simulink model "uz_3ph_ParameterID"  (R2022b)
settings: Solver=FixedStepDiscrete  StartTime=0.0  StopTime=160  FixedStep=0.000005  RelTol=1e-3  EnableMultiTasking=on
model workspace (MATLAB code in the model file):
  | cmdLim = Simulink.Parameter;
  | cmdLim.Value = 15;
  | cmdLim.Description = 'Limit for controlling the maximum surface command angle.';
  | cmdLim.Min = 0;
  | cmdLim.Max = 90;
  | cmdLim.DocUnits = 'deg';
  | 
  | dispGain = Simulink.Parameter;
  | dispGain.Value = 0.75;
  | dispGain.Description = 'Gain applied to the displacement error.';
  | dispGain.Min = 0;
  | dispGain.Max = [];
  | dispGain.DocUnits = 'deg/sec/deg';
  | 
  | dispLim = Simulink.Parameter;
  | dispLim.Value = 30;
  | dispLim.Description = 'Limit for controlling the maximum commanded angle.';
  | dispLim.Min = 0;
  | dispLim.Max = 180;
  | dispLim.DocUnits = 'deg';
  | 
  | intGain = Simulink.Parameter;
  | intGain.Value = 0.5;
  | intGain.Description = 'Gain applied to the integral error.';
  | intGain.Min = 0;
  | intGain.Max = [];
  | intGain.DocUnits = 'deg/sec/deg/sec';
  | 
  | intLim = Simulink.Parameter;
  | intLim.Value = 5;
  | intLim.Description = 'Limit for controlling the maximum commanded angle.';
  | intLim.Min = 0;
  | intLim.Max = 90;
  | intLim.DocUnits = 'deg';
  | 
  | rateGain = Simulink.Parameter;
  | rateGain.Value = 2;
  | rateGain.Description = 'Gain applied to the rate error.';
  | rateGain.Min = 0;
  | rateGain.Max = [];
  | rateGain.DocUnits = 'deg/deg/sec';
  | 
  | rateLim = Simulink.Parameter;
  | rateLim.Value = 6;
  | rateLim.Description = 'Limit for controlling the maximum commanded angle.';
  | rateLim.Min = 0;
  | rateLim.Max = 180;
  | rateLim.DocUnits = 'deg/sec';
  | 
  | hdgGain = Simulink.Parameter;
  | hdgGain.Value = 0.015;
values from neighbouring files (symbols this model uses):
  d_d_TMS = 0.005    [Parameter_Init_Buehler_201.m]
  d_f_hardware = 200000    [Parameter_Init_Buehler_201.m]
  d_f_states = 20000    [Parameter_Init_Buehler_201.m]
  d_i_max = 15    [Parameter_Init_Buehler_201.m]
  d_i_min = -d_i_max    (= -15)    [Parameter_Init_Buehler_201.m]
  d_I_n = 8    [Parameter_Init_Buehler_201.m]
  d_J_Coupling_M_E = 2e-6    (= 2e-06)    [Parameter_Init_Buehler_201.m]
  d_J_Coupling_M_Ms = 2e-20    [Parameter_Init_Buehler_201.m]
  d_J_Ms_L = d_J_Ms_M    (= 1.26363648e-05)    [Parameter_Init_Buehler_201.m]
  d_J_Ms_M = 0.5*0.5*((0.5*d_d_Ms)^4)*3.14*d_l_Ms*d_rho_Ms    (= 1.26363648e-05)    [Parameter_Init_Buehler_201.m]
  d_L_d = 0.00031    [Parameter_Init_Buehler_201.m]
  d_L_q = 0.00033    [Parameter_Init_Buehler_201.m]
  d_p = 4    [Parameter_Init_Buehler_201.m]
  d_psi_pm = 0.0075    [Parameter_Init_Buehler_201.m]
  d_R_ph = d_R_ph_ph/2    (= 0.089)    [Parameter_Init_Buehler_201.m]
  d_y_max = 10    [Parameter_Init_Buehler_201.m]
  d_y_min = -d_y_max    (= -10)    [Parameter_Init_Buehler_201.m]
undefined symbols (not defined in the file or in its folder): i_dq, i_dq_ref, n_ref, V_abc, v_dq
libraries: fl_lib x47, nesl_utility x30, ee_lib x18, simulink x8, spsabctodq0Lib x2, spsdq0toabcLib x1, spsTriangleGeneratorLib x1
(part 2 of 4)

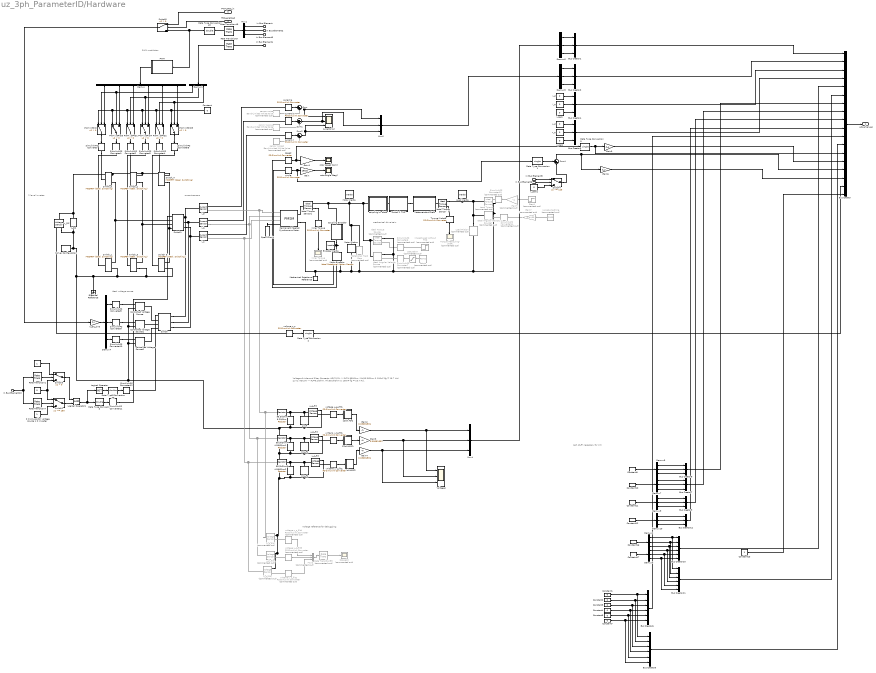
== system uz_3ph_ParameterID/Hardware ==
  note: 6ph stuff, necessary for init
  note: PWM modulator
  note: 2 level inverter
  note: current sensors
  note: ideal voltage source
  note: Voltage divider and filter:
      | Concerto: ADC 3,3V -> RL=4,99kOhm. Mit 95,3kOhm & 100nF (fg = 16,7 Hz).
      | Zynq: ADC 5V -> RL=8,2kOhm. Mit 95,3kOhm & 100nF (fg = 16,7 Hz).
  note: Voltage reference
      | for debugging:
  note: mechanical drive train
  In Bus Element : Inport  PortName=ElectricalID_output  Element=PWM_Switch_0
  In Bus Element2 : Inport  PortName=ElectricalID_output  Element=PWM_Switch_2
  In Bus Element3 : Inport  PortName=ElectricalID_output  Element=PWM_Switch_4
  In Bus Element4 : Inport  PortName=ElectricalID_output  Element=enable_TriState
  In Bus Element5 : Inport  PortName=ElectricalID_output  Element=thetaOffset
  In Bus Element10 : Inport  Port=2  PortName=ElectricalID_FOC_output  Element=activeState
  In Bus Element6 : Inport  Port=2  PortName=ElectricalID_FOC_output  Element=activeState
  PWM_FOC_in : Inport  Port=3
  FOC_enabled : Inport  Port=4
  " " : Constant  Value=0
  "   " : Constant
  "0 = sinusoidal voltage source 1 = inverter    " : Constant
  0.1µF1 : ee_lib/Passive/Capacitor  cap_option=0  c=47 nF  Cvec=[ 1e-5 1e-6 ] F  Vvec=[ 0 10 ] V  CV_table_symmetry=1  f_vec=[1, 10] kHz  DFext_vec=[.8, 1.2]  enable_C_tol=0  C_tol=0.1  tol_distribution=1  nSigma=4  r=1e-18 Ohm  g=0 1/Ohm  averaging_period=0 s  enable_operating_limits=0  operating_limit_action=2  max_working_voltage_range=[ -25 25 ] V  power_rating=1 W  enable_faults=0  fault_action=1  Cscale_faulted=100  R_faulted=0.001 Ohm  G_faulted=0 1/Ohm  tau_fault=0.001 s  enable_temporal_fault=0  t_fault=1 s  enable_behavioral_fault=0  max_permissible_voltage_range=[ -100 100 ] V  t_fail_on_voltage=1 s  i_specify=off  i_priority=None  i=0 A  i_nominal_specify=off  i_nominal_unit=A  i_nominal_value=1  v_specify=off  v_priority=None  v=0 V  v_nominal_specify=off  v_nominal_unit=V  v_nominal_value=1  vc_specify=on  vc_priority=High  vc=0 V  vc_nominal_specify=off  vc_nominal_unit=V  vc_nominal_value=1
  0.1µF2 : ee_lib/Passive/Capacitor  cap_option=0  c=47 nF  Cvec=[ 1e-5 1e-6 ] F  Vvec=[ 0 10 ] V  CV_table_symmetry=1  f_vec=[1, 10] kHz  DFext_vec=[.8, 1.2]  enable_C_tol=0  C_tol=0.1  tol_distribution=1  nSigma=4  r=1e-18 Ohm  g=0 1/Ohm  averaging_period=0 s  enable_operating_limits=0  operating_limit_action=2  max_working_voltage_range=[ -25 25 ] V  power_rating=1 W  enable_faults=0  fault_action=1  Cscale_faulted=100  R_faulted=0.001 Ohm  G_faulted=0 1/Ohm  tau_fault=0.001 s  enable_temporal_fault=0  t_fault=1 s  enable_behavioral_fault=0  max_permissible_voltage_range=[ -100 100 ] V  t_fail_on_voltage=1 s  i_specify=off  i_priority=None  i=0 A  i_nominal_specify=off  i_nominal_unit=A  i_nominal_value=1  v_specify=off  v_priority=None  v=0 V  v_nominal_specify=off  v_nominal_unit=V  v_nominal_value=1  vc_specify=on  vc_priority=High  vc=0 V  vc_nominal_specify=off  vc_nominal_unit=V  vc_nominal_value=1
  12bit ADC : MATLAB Function  TreatAsAtomicUnit=on
  12bit ADC1 : MATLAB Function  TreatAsAtomicUnit=on
  12bit ADC2 : MATLAB Function  TreatAsAtomicUnit=on
  4,99kOhm1 : ee_lib/Passive/Resistor  R=8200 Ohm  enable_R_tol=0  R_tol=0.1  tol_distribution=1  nSigma=4  enable_operating_limits=0  operating_limit_action=2  max_working_voltage=100 V  power_rating=1 W  enable_faults=0  fault_action=1  R_faulted=Inf Ohm  enable_temporal_fault=0  t_fault=1 s  enable_behavioral_fault=0  max_permissible_current=1 A  t_fail_on_current=1 s  noise_mode=0  sample_time=0.001 s  repeatability=1  auto_seed=3499211588  user_seed=0  Tdevice=25 degC  power_derating_T1=70 degC  power_derating_T2=155 degC  operating_temperature_range_vec=[-50, 150] degC  alpha=3.93e-3 1/K  Tmeas=25 degC  thermal_mass=100 J/K  temperature_specify=off  temperature_priority=High  temperature=298.15 K  temperature_nominal_specify=off  temperature_nominal_unit=K  temperature_nominal_value=1
  4,99kOhm2 : ee_lib/Passive/Resistor  R=8200 Ohm  enable_R_tol=0  R_tol=0.1  tol_distribution=1  nSigma=4  enable_operating_limits=0  operating_limit_action=2  max_working_voltage=100 V  power_rating=1 W  enable_faults=0  fault_action=1  R_faulted=Inf Ohm  enable_temporal_fault=0  t_fault=1 s  enable_behavioral_fault=0  max_permissible_current=1 A  t_fail_on_current=1 s  noise_mode=0  sample_time=0.001 s  repeatability=1  auto_seed=3890346746  user_seed=0  Tdevice=25 degC  power_derating_T1=70 degC  power_derating_T2=155 degC  operating_temperature_range_vec=[-50, 150] degC  alpha=3.93e-3 1/K  Tmeas=25 degC  thermal_mass=100 J/K  temperature_specify=off  temperature_priority=High  temperature=298.15 K  temperature_nominal_specify=off  temperature_nominal_unit=K  temperature_nominal_value=1
  47nF : ee_lib/Passive/Capacitor  cap_option=0  c=47 nF  Cvec=[ 1e-5 1e-6 ] F  Vvec=[ 0 10 ] V  CV_table_symmetry=1  f_vec=[1, 10] kHz  DFext_vec=[.8, 1.2]  enable_C_tol=0  C_tol=0.1  tol_distribution=1  nSigma=4  r=1e-20 Ohm  g=0 1/Ohm  averaging_period=0 s  enable_operating_limits=0  operating_limit_action=2  max_working_voltage_range=[ -25 25 ] V  power_rating=1 W  enable_faults=0  fault_action=1  Cscale_faulted=100  R_faulted=0.001 Ohm  G_faulted=0 1/Ohm  tau_fault=0.001 s  enable_temporal_fault=0  t_fault=1 s  enable_behavioral_fault=0  max_permissible_voltage_range=[ -100 100 ] V  t_fail_on_voltage=1 s  i_specify=off  i_priority=None  i=0 A  i_nominal_specify=off  i_nominal_unit=A  i_nominal_value=1  v_specify=off  v_priority=None  v=0 V  v_nominal_specify=off  v_nominal_unit=V  v_nominal_value=1  vc_specify=on  vc_priority=High  vc=0 V  vc_nominal_specify=off  vc_nominal_unit=V  vc_nominal_value=1
  8,2kOhm : ee_lib/Passive/Resistor  R=8200 Ohm  enable_R_tol=0  R_tol=0.1  tol_distribution=1  nSigma=4  enable_operating_limits=0  operating_limit_action=2  max_working_voltage=100 V  power_rating=1 W  enable_faults=0  fault_action=1  R_faulted=Inf Ohm  enable_temporal_fault=0  t_fault=1 s  enable_behavioral_fault=0  max_permissible_current=1 A  t_fail_on_current=1 s  noise_mode=0  sample_time=0.001 s  repeatability=1  auto_seed=545404223  user_seed=0  Tdevice=25 degC  power_derating_T1=70 degC  power_derating_T2=155 degC  operating_temperature_range_vec=[-50, 150] degC  alpha=3.93e-3 1/K  Tmeas=25 degC  thermal_mass=100 J/K  temperature_specify=off  temperature_priority=High  temperature=298.15 K  temperature_nominal_specify=off  temperature_nominal_unit=K  temperature_nominal_value=1
  95,3kOhm : ee_lib/Passive/Resistor  R=95300 Ohm  enable_R_tol=0  R_tol=0.1  tol_distribution=1  nSigma=4  enable_operating_limits=0  operating_limit_action=2  max_working_voltage=100 V  power_rating=1 W  enable_faults=0  fault_action=1  R_faulted=Inf Ohm  enable_temporal_fault=0  t_fault=1 s  enable_behavioral_fault=0  max_permissible_current=1 A  t_fail_on_current=1 s  noise_mode=0  sample_time=0.001 s  repeatability=1  auto_seed=3922919431  user_seed=0  Tdevice=25 degC  power_derating_T1=70 degC  power_derating_T2=155 degC  operating_temperature_range_vec=[-50, 150] degC  alpha=3.93e-3 1/K  Tmeas=25 degC  thermal_mass=100 J/K  temperature_specify=off  temperature_priority=High  temperature=298.15 K  temperature_nominal_specify=off  temperature_nominal_unit=K  temperature_nominal_value=1
  95,3kOhm4 : ee_lib/Passive/Resistor  R=95300 Ohm  enable_R_tol=0  R_tol=0.1  tol_distribution=1  nSigma=4  enable_operating_limits=0  operating_limit_action=2  max_working_voltage=100 V  power_rating=1 W  enable_faults=0  fault_action=1  R_faulted=Inf Ohm  enable_temporal_fault=0  t_fault=1 s  enable_behavioral_fault=0  max_permissible_current=1 A  t_fail_on_current=1 s  noise_mode=0  sample_time=0.001 s  repeatability=1  auto_seed=2715962282  user_seed=0  Tdevice=25 degC  power_derating_T1=70 degC  power_derating_T2=155 degC  operating_temperature_range_vec=[-50, 150] degC  alpha=3.93e-3 1/K  Tmeas=25 degC  thermal_mass=100 J/K  temperature_specify=off  temperature_priority=High  temperature=298.15 K  temperature_nominal_specify=off  temperature_nominal_unit=K  temperature_nominal_value=1
  95,3kOhm5 : ee_lib/Passive/Resistor  R=95300 Ohm  enable_R_tol=0  R_tol=0.1  tol_distribution=1  nSigma=4  enable_operating_limits=0  operating_limit_action=2  max_working_voltage=100 V  power_rating=1 W  enable_faults=0  fault_action=1  R_faulted=Inf Ohm  enable_temporal_fault=0  t_fault=1 s  enable_behavioral_fault=0  max_permissible_current=1 A  t_fail_on_current=1 s  noise_mode=0  sample_time=0.001 s  repeatability=1  auto_seed=418932850  user_seed=0  Tdevice=25 degC  power_derating_T1=70 degC  power_derating_T2=155 degC  operating_temperature_range_vec=[-50, 150] degC  alpha=3.93e-3 1/K  Tmeas=25 degC  thermal_mass=100 J/K  temperature_specify=off  temperature_priority=High  temperature=298.15 K  temperature_nominal_specify=off  temperature_nominal_unit=K  temperature_nominal_value=1
  Bus Creator : BusCreator  Inputs=18  OutDataTypeStr=Bus: uz_ParaID_ActualValues_t
  Bus Creator1 : BusCreator  Inputs=3  OutDataTypeStr=Bus: uz_3ph_abc_t
  Bus Creator10 : BusCreator  Inputs=6  OutDataTypeStr=Bus: uz_6ph_abc_t
  Bus Creator11 : BusCreator  Inputs=6  OutDataTypeStr=Bus: uz_6ph_abc_t
  Bus Creator{3..4,7..9,12} (6 alike) : BusCreator  Inputs=3  OutDataTypeStr=Bus: uz_3ph_dq_t
  Bus Creator2 : BusCreator  Inputs=3  OutDataTypeStr=Bus: uz_3ph_abc_t
  Bus Creator5 : BusCreator  Inputs=6  OutDataTypeStr=Bus: uz_6ph_dq_t
  Bus Creator6 : BusCreator  Inputs=6  OutDataTypeStr=Bus: uz_6ph_dq_t
  Constant : Constant  Value=0
  Constant{1..5,7} (6 alike) : Constant  Value=0  OutDataTypeStr=single
  Constant{9..12,16..17} (6 alike) : Constant  Value=[0;0;0]  OutDataTypeStr=single
  Constant13 : Constant  OutDataTypeStr=single
  Controlled Voltage Source : fl_lib/Electrical/Electrical Sources/Controlled Voltage Source
  Controlled Voltage Source1 : fl_lib/Electrical/Electrical Sources/Controlled Voltage Source
  Controlled Voltage Source2 : fl_lib/Electrical/Electrical Sources/Controlled Voltage Source
  Coupling Encoder : Subsystem  Variant=on  VariantControlMode=label  LabelModeActiveChoice=TMS1
  Data Type Conversion1 : DataTypeConversion  OutDataTypeStr=single  SaturateOnIntegerOverflow=off  RndMeth=Floor
  Data Type Conversion2 : DataTypeConversion  OutDataTypeStr=single  SaturateOnIntegerOverflow=off  RndMeth=Floor
  Data Type Conversion3 : DataTypeConversion  OutDataTypeStr=double  SaturateOnIntegerOverflow=off  RndMeth=Floor
  Data Type Conversion48 : DataTypeConversion  OutDataTypeStr=double  SaturateOnIntegerOverflow=off  RndMeth=Floor
  Data Type Conversion49 : DataTypeConversion  OutDataTypeStr=double  SaturateOnIntegerOverflow=off  RndMeth=Floor
  Data Type Conversion5 : DataTypeConversion  OutDataTypeStr=single  SaturateOnIntegerOverflow=off  RndMeth=Floor
  Demux : Demux  Outputs=6
  Demux{1..10} (10 alike) : Demux  Outputs=3
  Electrical Reference : fl_lib/Electrical/Electrical Elements/Electrical Reference
  Encoder Inertia : fl_lib/Mechanical/Rotational Elements/Inertia  inertia=d_J_Encoder kg*m^2  num_ports=foundation.enum.numPorts2.one  w_specify=off  w_priority=High  w=0 rad/s  w_nominal_specify=off  w_nominal_unit=rad/s  w_nominal_value=1  t_specify=off  t_priority=None  t=0 N*m  t_nominal_specify=off  t_nominal_unit=N*m  t_nominal_value=1
  Gain : Gain  Gain=180/pi
  Gain1 : Gain  Gain=60/(2*pi)
  Gain2 : Gain  Gain=0.03081531  OutDataTypeStr=single
  Gain3 : Gain  Gain=0.03081531  OutDataTypeStr=single
  Gain4 : Gain  Gain=0.03081531  OutDataTypeStr=single
  Gain5 : Gain  Commented=on  Gain=-1
  Gain6 : Gain  Gain=d_p  OutDataTypeStr=single
  Gain7 : Gain  Commented=on  Gain=2*pi/60
  Gain9 : Gain  Gain=d_p  OutDataTypeStr=single
  Ideal Angular Velocity Source : fl_lib/Mechanical/Mechanical Sources/Ideal Angular Velocity Source  Commented=on
  Ideal Angular Velocity Source1 : fl_lib/Mechanical/Mechanical Sources/Ideal Angular Velocity Source  Commented=on
  Ideal Torque Sensor : fl_lib/Mechanical/Mechanical Sensors/Ideal Torque Sensor
  Ideal Torque Sensor1 : fl_lib/Mechanical/Mechanical Sensors/Ideal Torque Sensor
  Ideal Torque Source : fl_lib/Mechanical/Mechanical Sources/Ideal Torque Source  Commented=on
  Impact Load without TMS : Step  Commented=on  Time=0.05  SampleTime=1/d_f_states
  Inner Torque : nesl_utility/PS-Simulink Converter  PhysicalDomain=network_engine_domain  SubClassName=ps_output  LeftPortType=input  RightPortType=output  PseudoPeriodic=off  Frequencies=[]  VectorFormat=1-D array  Unit=N*m  AffineConversion=off
  "Inner Torque " : Scope  Commented=on
  Load Friction : fl_lib/Mechanical/Rotational Elements/Rotational Friction  Commented=on  brkwy_trq=d_M_stribeck N*m  brkwy_vel=d_v_stribeck rad/s  Col_trq=d_M_coulomb N*m  visc_coef=d_d_viscous N*m/(rad/s)  w_specify=on  w_priority=High  w=0 rad/s  w_nominal_specify=off  w_nominal_unit=rad/s  w_nominal_value=1  t_specify=on  t_priority=High  t=0 N*m  t_nominal_specify=off  t_nominal_unit=N*m  t_nominal_value=1
  Load Inertia : fl_lib/Mechanical/Rotational Elements/Inertia  inertia=d_J_Loadmachine kg*m^2  num_ports=foundation.enum.numPorts2.one  w_specify=off  w_priority=High  w=0 rad/s  w_nominal_specify=off  w_nominal_unit=rad/s  w_nominal_value=1  t_specify=off  t_priority=None  t=0 N*m  t_nominal_specify=off  t_nominal_unit=N*m  t_nominal_value=1
  Load Torque : fl_lib/Mechanical/Mechanical Sources/Ideal Torque Source  Commented=on
  Logical Operator : Logic  Operator=NOT  AllPortsSameDT=off  OutDataTypeStr=boolean
  Logical Operator1 : Logic  AllPortsSameDT=off  OutDataTypeStr=boolean
  Measurement Shaft : Subsystem  Variant=on  VariantControlMode=label  LabelModeActiveChoice=TMS1
  Mechanical Rotational Reference : fl_lib/Mechanical/Rotational Elements/Mechanical Rotational Reference
  Motor Encoder : fl_lib/Mechanical/Mechanical Sensors/Ideal Rotational Motion Sensor  reference=foundation.enum.MeasurementReference.difference  acceleration_port=false  velocity_port=true  position_port=true  wrap_angle=simscape.enum.onoff.off  offset=0 deg
  "Motor Inertia " : fl_lib/Mechanical/Rotational Elements/Inertia  inertia=d_J_m kg*m^2  num_ports=foundation.enum.numPorts2.one  w_specify=off  w_priority=High  w=0 rad/s  w_nominal_specify=off  w_nominal_unit=rad/s  w_nominal_value=1  t_specify=off  t_priority=None  t=0 N*m  t_nominal_specify=off  t_nominal_unit=N*m  t_nominal_value=1
  Motor Friction : fl_lib/Mechanical/Rotational Elements/Rotational Friction  brkwy_trq=d_M_stribeck N*m  brkwy_vel=d_v_stribeck rad/s  Col_trq=d_M_coulomb N*m  visc_coef=d_d_viscous N*m/(rad/s)  w_specify=on  w_priority=High  w=0 rad/s  w_nominal_specify=off  w_nominal_unit=rad/s  w_nominal_value=1  t_specify=on  t_priority=High  t=0 N*m  t_nominal_specify=off  t_nominal_unit=N*m  t_nominal_value=1
  Mux1 : Mux  Inputs=3
  Mux2 : Mux  Commented=on  Inputs=3
  Mux4 : Mux  Inputs=3
  Mux6 : Mux  Inputs=3
  Open Circuit : fl_lib/Electrical/Electrical Elements/Open Circuit  v_specify=off  v_priority=None  v=0 V  v_nominal_specify=off  v_nominal_unit=V  v_nominal_value=1
  PWM : Subsystem
  PWM | GPIO{,1..5} (6 alike) : Switch  Criteria=u2 > Threshold  SaturateOnIntegerOverflow=off  InputSameDT=off
  Permanent Magnet Synchronous Motor : ee_lib/Electromechanical/Permanent Magnet/PMSM  port_option=ee.enum.threePhasePort.expanded  winding_type=ee.enum.statorconnection.wye  machine_param=ee.enum.pmsm.parameterization.constant  nPolePairs=d_p  pmflux_param=1  pm_flux_linkage=d_psi_pm Wb  torque_constant=0.18 N*m/A  back_emf_constant=0.18 V/(rad/s)  stator_param=1  Ld=d_L_d H  Lq=d_L_q H  idVec=[-200, 0, 200] A  iqVec=[-200, 0, 200] A  LdMatrix=0.0002 * ones(3, 3) H  LqMatrix=0.0002 * ones(3, 3) H  PmMatrix=0.1 * ones(3, 3) Wb  ktMatrix=0.18 * ones(3, 3) N*m/A  keMatrix=0.18 * ones(3, 3) V/(rad/s)  L0=d_L_0 H  Ls=0.0002 H  Lm=0.00002 H  Ms=0.00002 H  Rs=d_R_ph Ohm  zero_sequence=ee.enum.park.zerosequence.include  axes_param=2  loss_param=ee.enum.ironloss.none  losses_oc=[0, 0, 0] W  losses_sc=[0, 0, 0] W  f_losses=60 Hz  Isc_losses=95 A  J=0 kg*m^2  lam=0 N*m/(rad/s)  i_d_specify=off  i_d_priority=None  i_d=0 A  i_d_nominal_specify=off  i_d_nominal_unit=A  i_d_nominal_value=1  i_q_specify=off  i_q_priority=None  i_q=0 A  i_q_nominal_specify=off  i_q_nominal_unit=A  i_q_nominal_value=1  torque_specify=off  torque_priority=None  torque=0 N*m  torque_nominal_specify=off  torque_nominal_unit=N*m  torque_nominal_value=1  angular_velocity_specify=on  angular_velocity_priority=None  angular_velocity=0 rpm  angular_velocity_nominal_specify=off  angular_velocity_nominal_unit=rpm  angular_velocity_nominal_value=1  angular_position_specify=on  angular_position_priority=High  angular_position=0 deg  angular_position_nominal_specify=off  angular_position_nominal_unit=deg  angular_position_nominal_value=1  alpha=3.93e-3 1/K  alpha_flux=-0.001 1/K  Tmeas=298.15 K  stator_thermal_mass=100 J/K  rotor_thermal_mass=200 J/K  Rm_percent_rotor=90  Rd_percent_rotor=30  temperatureA_specify=off  temperatureA_priority=High  temperatureA=25 degC  temperatureA_nominal_specify=off  temperatureA_nominal_unit=degC  temperatureA_nominal_value=1  temperatureB_specify=off  temperatureB_priority=High  temperatureB=25 degC  temperatureB_nominal_specify=off  temperatureB_nominal_unit=degC  temperatureB_nominal_value=1  temperatureC_specify=off  temperatureC_priority=High  temperatureC=25 degC  temperatureC_nominal_specify=off  temperatureC_nominal_unit=degC  temperatureC_nominal_value=1  temperatureR_specify=off  temperatureR_priority=High  temperatureR=25 degC  temperatureR_nominal_specify=off  temperatureR_nominal_unit=degC  temperatureR_nominal_value=1
      settings: InternalSimscapePortConfiguration="{\"Bottom\":[],\"Left\":[{\"id\":\"a\",\"label\":\"a\",\"type\":\"foundation.electrical.electrical\"},{\"id\":\"b\",\"label\":\"b\",\"type\":\"foundation.electrical.electrical\"},{\"id\":\"c\",\"label\":\"c\",\"type\":\"foundation.electrical.electrical\"},{\"id\":\"n\",\"label\":\"n\",\"type\":\"foundation.electrical.electrical\"}],\"Right\":[{\"id\":\"R\",\"label\":\"R\",\"type\":\"foundation.mechanical.rotational.rotational\"},{\"id\":\"C\",\"label\":\"C\",\"type\":\"foundation.mechanical.rotational.rotational\"}],\"Top\":[]}"
  Ramp : simulink/Sources/Ramp  Commented=on  slope=10000  start=0  InitialOutput=0
  Rate Transition{1,7,9,45} (4 alike) : RateTransition  OutPortSampleTime=1/d_f_hardware
  Rate Transition55 : RateTransition  Commented=on  OutPortSampleTime=1/d_f_states
  Rotational Hard Stop : fl_lib/Mechanical/Rotational Elements/Rotational Hard Stop  Commented=on  upper_bnd=999999 rad  lower_bnd=0 rad  stiff_up=1e6 N*m/rad  stiff_low=1e6 N*m/rad  D_up=0.01 N*m/(rad/s)  D_low=0.01 N*m/(rad/s)  model=3  transition=0.001 rad  w_specify=off  w_priority=None  w=0 rad/s  w_nominal_specify=off  w_nominal_unit=rad/s  w_nominal_value=1  t_specify=off  t_priority=None  t=0 N*m  t_nominal_specify=off  t_nominal_unit=N*m  t_nominal_value=1  phi_specify=off  phi_priority=High  phi=0 rad  phi_nominal_specify=off  phi_nominal_unit=rad  phi_nominal_value=1
  Saturation : Saturate  Commented=on  UpperLimit=104.7/2
  Scope10 : Scope  Commented=on
  Simulink-PS Converter{,1..5,8..12} (11 alike) : nesl_utility/Simulink-PS Converter  PhysicalDomain=network_engine_domain  SubClassName=ps_input  LeftPortType=input  RightPortType=output  PseudoPeriodic=off  Frequencies=[]  NoiseDistribution=none  NoiseParameters=[]  Unit=1  AffineConversion=off  FilteringAndDerivatives=zero  SimscapeFilterOrder=1  InputFilterTimeConstant=0.001  UdotUserProvided=1
  Simulink-PS Converter13 : nesl_utility/Simulink-PS Converter  Commented=on  PhysicalDomain=network_engine_domain  SubClassName=ps_input  LeftPortType=input  RightPortType=output  PseudoPeriodic=off  Frequencies=[]  NoiseDistribution=none  NoiseParameters=[]  Unit=1  AffineConversion=off  FilteringAndDerivatives=zero  SimscapeFilterOrder=1  InputFilterTimeConstant=0.001  UdotUserProvided=1
  Simulink-PS Converter14 : nesl_utility/Simulink-PS Converter  Commented=on  PhysicalDomain=network_engine_domain  SubClassName=ps_input  LeftPortType=input  RightPortType=output  PseudoPeriodic=off  Frequencies=[]  NoiseDistribution=none  NoiseParameters=[]  Unit=1  AffineConversion=off  FilteringAndDerivatives=zero  SimscapeFilterOrder=1  InputFilterTimeConstant=0.001  UdotUserProvided=1
  Simulink-PS Converter6 : nesl_utility/Simulink-PS Converter  Commented=on  PhysicalDomain=network_engine_domain  SubClassName=ps_input  LeftPortType=input  RightPortType=output  PseudoPeriodic=off  Frequencies=[]  NoiseDistribution=none  NoiseParameters=[]  Unit=N*m  AffineConversion=off  FilteringAndDerivatives=zero  SimscapeFilterOrder=1  InputFilterTimeConstant=0.001  UdotUserProvided=1
  Simulink-PS Converter7 : nesl_utility/Simulink-PS Converter  Commented=on  PhysicalDomain=network_engine_domain  SubClassName=ps_input  LeftPortType=input  RightPortType=output  PseudoPeriodic=off  Frequencies=[]  NoiseDistribution=none  NoiseParameters=[]  Unit=rad/s  AffineConversion=off  FilteringAndDerivatives=zero  SimscapeFilterOrder=1  InputFilterTimeConstant=0.001  UdotUserProvided=1
  Solver Configuration : nesl_utility/Solver Configuration  PhysicalDomain=network_engine_domain  SubClassName=solver  LeftPortType=input  RightPortType=generic  Tones=[]  Harmonics=[]  SimulateNoise=off  Profile=off  UseLocalSampling=off  EnableSwitchedLinearOptims=on  FrequencyDomain=off  UseCCode=off  RelTol=0.001  AbsTol=1e-06  MinStep=1e-09  ToWorkspace=off  RevertToSquareIcSolve=off  NumHomotopyIterations=100  PhasorMode=off  PhasorModeNumHarmonics=1  ConsistencySolver=NEWTON_FTOL  IndexReductionMethod=DerivativeReplacement  DoDC=off  ResidualTolerance=1e-09  ConsistencyTolSource=GLOBAL  ConsistencyAbsTol=0.001  ConsistencyRelTol=0.001  ConsistencyTolFactor=0.001  UseLocalSolver=on  LocalSolverChoice=NE_BACKWARD_EULER_ADVANCER  ResolveIndetEquations=on  FunctionEvalNumThread=1  LocalSolverSampleTime=1/d_f_hardware  DoFixedCost=on  MaxNonlinIter=3  MaxModeIter=2  ComputeImpulses=off  ImpulseIterations=2  LinearAlgebra=Sparse  LinearAlgebraNumThread=0  EquationFormulation=NE_TIME_EF  DelaysMemoryBudget=1024  AutomaticFiltering=on  FilteringTimeConstant=0.001  PartitionStorageMethod=AS_NEEDED  PartitionMemoryBudget=1024  PartitionMethod=FAST
  Step1 : Step  Commented=on  Time=0  After=0.3  SampleTime=0
  Sum : Sum  Inputs=|++  OutDataTypeStr=single
  Sum1 : Sum  Inputs=|++  OutDataTypeStr=single
  Sum2 : Sum  Inputs=|++  OutDataTypeStr=single
  Sum4 : Sum  Inputs=+-|
  Switch : ee_lib/Switches & Breakers/SPST Switch (Three-Phase)  R_closed=0.001 Ohm  G_open=1e-6 1/Ohm  threshold=0.1 V  i_vT_specify=off  i_vT_priority=None  i_vT=0 A  i_vT_nominal_specify=off  i_vT_nominal_unit=A  i_vT_nominal_value=1  I_specify=off  I_priority=None  I=[ 0 0 0 ] A  I_nominal_specify=off  I_nominal_unit=A  I_nominal_value=1  V_specify=off  V_priority=None  V=[ 0 0 0 ] V  V_nominal_specify=off  V_nominal_unit=V  V_nominal_value=1  i_a_specify=off  i_a_priority=None  i_a=0 A  i_a_nominal_specify=off  i_a_nominal_unit=A  i_a_nominal_value=1  v_a_specify=off  v_a_priority=None  v_a=0 V  v_a_nominal_specify=off  v_a_nominal_unit=V  v_a_nominal_value=1  i_b_specify=off  i_b_priority=None  i_b=0 A  i_b_nominal_specify=off  i_b_nominal_unit=A  i_b_nominal_value=1  v_b_specify=off  v_b_priority=None  v_b=0 V  v_b_nominal_specify=off  v_b_nominal_unit=V  v_b_nominal_value=1  i_c_specify=off  i_c_priority=None  i_c=0 A  i_c_nominal_specify=off  i_c_nominal_unit=A  i_c_nominal_value=1  v_c_specify=off  v_c_priority=None  v_c=0 V  v_c_nominal_specify=off  v_c_nominal_unit=V  v_c_nominal_value=1
      settings: InternalSimscapePortConfiguration="{\"Bottom\":[],\"Left\":[{\"id\":\"vT\",\"label\":\"vT\",\"type\":\"input\"},{\"id\":\"a1\",\"label\":\"a1\",\"type\":\"foundation.electrical.electrical\"},{\"id\":\"b1\",\"label\":\"b1\",\"type\":\"foundation.electrical.electrical\"},{\"id\":\"c1\",\"label\":\"c1\",\"type\":\"foundation.electrical.electrical\"}],\"Right\":[{\"id\":\"a2\",\"label\":\"a2\",\"type\":\"foundation.electrical.electrical\"},{\"id\":\"b2\",\"label\":\"b2\",\"type\":\"foundation.electrical.electrical\"},{\"id\":\"c2\",\"label\":\"c2\",\"type\":\"foundation.electrical.electrical\"}],\"Top\":[]}"
  Switch f. TMS : Subsystem  Variant=on  VariantControlMode=label  LabelModeActiveChoice=d_KupplZus==1
  Switch1 : ee_lib/Switches & Breakers/SPST Switch (Three-Phase)  R_closed=0.001 Ohm  G_open=1e-6 1/Ohm  threshold=0.1 V  i_vT_specify=off  i_vT_priority=None  i_vT=0 A  i_vT_nominal_specify=off  i_vT_nominal_unit=A  i_vT_nominal_value=1  I_specify=off  I_priority=None  I=[ 0 0 0 ] A  I_nominal_specify=off  I_nominal_unit=A  I_nominal_value=1  V_specify=off  V_priority=None  V=[ 0 0 0 ] V  V_nominal_specify=off  V_nominal_unit=V  V_nominal_value=1  i_a_specify=off  i_a_priority=None  i_a=0 A  i_a_nominal_specify=off  i_a_nominal_unit=A  i_a_nominal_value=1  v_a_specify=off  v_a_priority=None  v_a=0 V  v_a_nominal_specify=off  v_a_nominal_unit=V  v_a_nominal_value=1  i_b_specify=off  i_b_priority=None  i_b=0 A  i_b_nominal_specify=off  i_b_nominal_unit=A  i_b_nominal_value=1  v_b_specify=off  v_b_priority=None  v_b=0 V  v_b_nominal_specify=off  v_b_nominal_unit=V  v_b_nominal_value=1  i_c_specify=off  i_c_priority=None  i_c=0 A  i_c_nominal_specify=off  i_c_nominal_unit=A  i_c_nominal_value=1  v_c_specify=off  v_c_priority=None  v_c=0 V  v_c_nominal_specify=off  v_c_nominal_unit=V  v_c_nominal_value=1
      settings: InternalSimscapePortConfiguration="{\"Bottom\":[],\"Left\":[{\"id\":\"vT\",\"label\":\"vT\",\"type\":\"input\"},{\"id\":\"a1\",\"label\":\"a1\",\"type\":\"foundation.electrical.electrical\"},{\"id\":\"b1\",\"label\":\"b1\",\"type\":\"foundation.electrical.electrical\"},{\"id\":\"c1\",\"label\":\"c1\",\"type\":\"foundation.electrical.electrical\"}],\"Right\":[{\"id\":\"a2\",\"label\":\"a2\",\"type\":\"foundation.electrical.electrical\"},{\"id\":\"b2\",\"label\":\"b2\",\"type\":\"foundation.electrical.electrical\"},{\"id\":\"c2\",\"label\":\"c2\",\"type\":\"foundation.electrical.electrical\"}],\"Top\":[]}"
  Switch2 : Switch  Threshold=150  SaturateOnIntegerOverflow=off  InputSameDT=off
  Switch3 : Switch  Criteria=u2 > Threshold  SaturateOnIntegerOverflow=off  InputSameDT=off
  Switch4 : Switch  Threshold=125  SaturateOnIntegerOverflow=off  InputSameDT=off
  Switch5 : Switch  Criteria=u2 > Threshold  SaturateOnIntegerOverflow=off  InputSameDT=off
  Switch_{0..5} (6 alike) : ee_lib/Semiconductors & Converters/MOSFET (Ideal, Switching)  port_option=ee.enum.controlport.ps  Rds=0.0077 Ohm  Goff=1e-6 1/Ohm  Vth=0.2 V  diode_param=2  diode_Vf=0.8 V  diode_Ron=0.001 Ohm  diode_Goff=1e-5 1/Ohm  diode_C=5e-8 F  diode_iRM=-235 A  diode_iF=300 A  diode_idot=-50 A/us  diode_trr_param=1  diode_trr_factor=3  diode_trr=15 us  diode_Qrr=1.5e+3 s*uA  ids_specify=off  ids_priority=None  ids=0 A  ids_nominal_specify=off  ids_nominal_unit=A  ids_nominal_value=1  vds_specify=off  vds_priority=None  vds=0 V  vds_nominal_specify=off  vds_nominal_unit=V  vds_nominal_value=1  vgs_specify=off  vgs_priority=None  vgs=0 V  vgs_nominal_specify=off  vgs_nominal_unit=V  vgs_nominal_value=1  thermal_loss_option=ee.enum.converters.thermalLossOption.constantvalues  Von_data=[0, 1.8, 3.2, 6, 10, 16; 0, 2, 5.5, 9.5, 15, 25] V  Tj=[298.15, 448.15] K  Iout_data=[0, 20, 40, 60, 80, 100] A  Eon_data=[0, 55.04, 124.57, 235.53, 362.12; 0, 71.25, 161.25, 304.88, 468.75] * 1e-6 J  Eoff_data=[0, 18, 30, 56.1, 76.5; 0, 22.5, 37.5, 70.13, 95.63] * 1e-6 J  Tj_loss=[298.15, 448.15] K  Iout_data_loss=[0, 10, 20, 30, 40] A  Eon_scalar=22.86e-3 J  Eoff_scalar=17.14e-3 J  Voff=300 V  Iout_scalar=600 A  diodeModelType=ee.enum.converters.diodeModelType.pwl  diodeTableType=ee.enum.diode.tableType.IfMat  diode_IfMat=[.07, .12, .19, 1.75, 4.24, 7.32, 11.2; .16, .3, .72, 2.14, 4.02, 6.35, 9.12] A  diode_VfMat=[.9, 1.15, 1.25, 1.5, 1.75, 2.17, 2.6, 2.85; .58, .68, .75, 1.1, 1.38, 1.77, 2.27, 2.7] V  diode_TjVec=[25, 125] degC  diode_VfVec=[.5, .7, .9, 1.3, 1.7, 2.1, 2.5] V  diode_IfVec=[.1, .2, .5, 1, 2, 4, 7, 10] A  diode_Vr=-600 V  diode_Ls=150 nH  diode_Erec=0.03 J  thermal_network_parameterization=ee.enum.thermalNetworkTopology.external  Rth=[.03, .2] K/W  Rth_Cauer=[.03, .1, .2] K/W  Rth_Foster=[.03, .2] K/W  thermal_mass_parameterization=ee.enum.thermalNetwork.timeconstant  thermal_mass=[3, 25] J/K  thermal_mass_Cauer=[3, 10, 25] J/K  thermal_mass_Foster=[33, 50] J/K  thermal_time_constant=[.1, 5] s  thermal_time_constant_Cauer=[.1, 1, 5] s  thermal_time_constant_Foster=[1, 10] s  thermal_mass_initial_temperatures=[25, 25] degC  thermal_mass_initial_temperatures_Cauer=[25, 25, 25] degC  junction_thermal_mass=0.1 J/K  Tvec_initial_Foster=[25, 25, 25, 25] degC  no_thermal_network=0  junction_temperature_specify=off  junction_temperature_priority=None  junction_temperature=25 degC  junction_temperature_nominal_specify=off  junction_temperature_nominal_unit=degC  junction_temperature_nominal_value=1  Qj_specify=off  Qj_priority=None  Qj=0 W  Qj_nominal_specify=off  Qj_nominal_unit=W  Qj_nominal_value=1
  Torque Measuring- shaft : Scope  Commented=on
  Torque M.shaft : nesl_utility/PS-Simulink Converter  PhysicalDomain=network_engine_domain  SubClassName=ps_output  LeftPortType=input  RightPortType=output  PseudoPeriodic=off  Frequencies=[]  VectorFormat=1-D array  Unit=N*m  AffineConversion=off
  V_DC : fl_lib/Electrical/Electrical Sources/DC Voltage Source  v0=V_DC V
  V_DC_sine : Gain  Gain=24
  Voltages : Scope  NumInputPorts=3
  angle : nesl_utility/PS-Simulink Converter  PhysicalDomain=network_engine_domain  SubClassName=ps_output  LeftPortType=input  RightPortType=output  PseudoPeriodic=off  Frequencies=[]  VectorFormat=1-D array  Unit=rad  AffineConversion=off
  coupling m. shaft : Subsystem  Variant=on  VariantControlMode=label  LabelModeActiveChoice=TMS1
  current a : nesl_utility/PS-Simulink Converter  PhysicalDomain=network_engine_domain  SubClassName=ps_output  LeftPortType=input  RightPortType=output  PseudoPeriodic=off  Frequencies=[]  VectorFormat=1-D array  Unit=A  AffineConversion=off
  current b : nesl_utility/PS-Simulink Converter  PhysicalDomain=network_engine_domain  SubClassName=ps_output  LeftPortType=input  RightPortType=output  PseudoPeriodic=off  Frequencies=[]  VectorFormat=1-D array  Unit=A  AffineConversion=off
  current c : nesl_utility/PS-Simulink Converter  PhysicalDomain=network_engine_domain  SubClassName=ps_output  LeftPortType=input  RightPortType=output  PseudoPeriodic=off  Frequencies=[]  VectorFormat=1-D array  Unit=A  AffineConversion=off
  currents [A] : Scope  NumInputPorts=3
  i_a : fl_lib/Electrical/Electrical Sensors/Current Sensor
  i_b : fl_lib/Electrical/Electrical Sensors/Current Sensor
  i_c : fl_lib/Electrical/Electrical Sensors/Current Sensor
  i_d : Constant  Value=0  OutDataTypeStr=single
  i_q : Constant  Value=0  OutDataTypeStr=single
  i_zero : Constant  Value=0  OutDataTypeStr=single
  n_load_machine : Constant  Commented=on  Value=1000
  rotor angle [deg] : Scope
  rotor speed [rpm] : Scope
  sensor noise : simulink/Sources/Band-Limited White Noise  Commented=on  Cov=[0.0000000001]  Ts=1/d_f_hardware  seed=[23341]
  sensor noise1 : simulink/Sources/Band-Limited White Noise  Commented=on  Cov=[0.0000000001]  Ts=1/d_f_hardware  seed=[43132]
  sensor noise2 : simulink/Sources/Band-Limited White Noise  Commented=on  Cov=[0.0000000001]  Ts=1/d_f_hardware  seed=[12334]
  speed : nesl_utility/PS-Simulink Converter  PhysicalDomain=network_engine_domain  SubClassName=ps_output  LeftPortType=input  RightPortType=output  PseudoPeriodic=off  Frequencies=[]  VectorFormat=1-D array  Unit=rad/s  AffineConversion=off
  u_a_filt : fl_lib/Electrical/Electrical Sensors/Voltage Sensor
      settings: LogSimulationData=on
  u_a_filt1 : fl_lib/Electrical/Electrical Sensors/Voltage Sensor  Commented=on
      settings: LogSimulationData=on
  u_b_filt : fl_lib/Electrical/Electrical Sensors/Voltage Sensor
      settings: LogSimulationData=on
  u_b_filt1 : fl_lib/Electrical/Electrical Sensors/Voltage Sensor  Commented=on
      settings: LogSimulationData=on
  u_c_filt : fl_lib/Electrical/Electrical Sensors/Voltage Sensor
      settings: LogSimulationData=on
  u_c_filt1 : fl_lib/Electrical/Electrical Sensors/Voltage Sensor  Commented=on
      settings: LogSimulationData=on
  v_DC : fl_lib/Electrical/Electrical Sensors/Voltage Sensor
  v_d : Constant  Value=0  OutDataTypeStr=single
  v_q : Constant  Value=0  OutDataTypeStr=single
  v_zero : Constant  Value=0  OutDataTypeStr=single
  v_zero1 : Constant  Value=0  OutDataTypeStr=single
  voltage u_a_filt1 : nesl_utility/PS-Simulink Converter  PhysicalDomain=network_engine_domain  SubClassName=ps_output  LeftPortType=input  RightPortType=output  PseudoPeriodic=off  Frequencies=[]  VectorFormat=1-D array  Unit=V  AffineConversion=off
  voltage u_b_filt1 : nesl_utility/PS-Simulink Converter  PhysicalDomain=network_engine_domain  SubClassName=ps_output  LeftPortType=input  RightPortType=output  PseudoPeriodic=off  Frequencies=[]  VectorFormat=1-D array  Unit=V  AffineConversion=off
  voltage u_c_filt1 : nesl_utility/PS-Simulink Converter  PhysicalDomain=network_engine_domain  SubClassName=ps_output  LeftPortType=input  RightPortType=output  PseudoPeriodic=off  Frequencies=[]  VectorFormat=1-D array  Unit=V  AffineConversion=off
  voltage u_c_filt2 : nesl_utility/PS-Simulink Converter  Commented=on  PhysicalDomain=network_engine_domain  SubClassName=ps_output  LeftPortType=input  RightPortType=output  PseudoPeriodic=off  Frequencies=[]  VectorFormat=1-D array  Unit=V  AffineConversion=off
  voltage u_c_filt3 : nesl_utility/PS-Simulink Converter  Commented=on  PhysicalDomain=network_engine_domain  SubClassName=ps_output  LeftPortType=input  RightPortType=output  PseudoPeriodic=off  Frequencies=[]  VectorFormat=1-D array  Unit=V  AffineConversion=off
  voltage u_c_filt4 : nesl_utility/PS-Simulink Converter  Commented=on  PhysicalDomain=network_engine_domain  SubClassName=ps_output  LeftPortType=input  RightPortType=output  PseudoPeriodic=off  Frequencies=[]  VectorFormat=1-D array  Unit=V  AffineConversion=off
  voltage u_s : nesl_utility/PS-Simulink Converter  PhysicalDomain=network_engine_domain  SubClassName=ps_output  LeftPortType=input  RightPortType=output  PseudoPeriodic=off  Frequencies=[]  VectorFormat=1-D array  Unit=V  AffineConversion=off
  ActualValues : Outport
  wires:
  Demux/2 -> PWM | GPIO3/3
  sensor noise1/1 -> Sum1/2
  Demux/3 -> PWM | GPIO1/3
  Demux1/3 -> PWM | GPIO5/2, PWM | GPIO2/2
  Gain/1 -> rotor angle [deg]/1  "rotor angle"
  Rate Transition9/1 -> Demux1/1
  Demux/4 -> PWM | GPIO4/3
  V_DC_sine/1 -> Demux4/1
  Torque M.shaft/1 -> Torque Measuring- shaft/1
  Switch5/1 -> V_DC_sine/1
  Sum/1 -> currents [A]/1, Mux6/1  "i_a"
  voltage u_a_filt1/1 -> 12bit ADC/1(u)
  Gain3/1 -> Voltages/2, Mux4/2  "u_b"
  PWM/1(Out1) -> Demux/1
  Demux/1 -> PWM | GPIO/3
  current b/1 -> Sum1/1
  Demux1/1 -> PWM | GPIO3/2, PWM | GPIO/2
  PWM | GPIO4/1 -> Simulink-PS Converter3/1
  Data Type Conversion2/1 -> Bus Creator/17  "V_DC"
  PWM | GPIO5/1 -> Simulink-PS Converter5/1
  Demux1/2 -> PWM | GPIO4/2, PWM | GPIO1/2
  Mux1/1 -> Rate Transition45/1
  current a/1 -> Sum/1
  Sum2/1 -> Mux6/3, currents [A]/3  "i_c"
  sensor noise/1 -> Sum/2
  Step1/1 -> Gain5/1
  Gain1/1 -> rotor speed [rpm]/1  "rotor speed"
  PWM | GPIO1/1 -> Simulink-PS Converter2/1
  Logical Operator/1 -> Data Type Conversion49/1
  current c/1 -> Sum2/1
  Demux/6 -> PWM | GPIO5/3
  Gain7/1 -> Simulink-PS Converter14/1
  Sum1/1 -> currents [A]/2, Mux6/2  "i_b"
  speed/1 -> Data Type Conversion5/1, Gain1/1  "omega_m"
  Demux/5 -> PWM | GPIO2/3
  Gain2/1 -> Voltages/1, Mux4/1  "u_a"
  12bit ADC/1(y) -> Gain2/1
  Rate Transition55/1 -> Scope10/1
  Mux6/1 -> Demux8/1  "V_UVW"
  Sum4/1 -> Bus Creator/15, Gain6/1  "theta_m"
  voltage u_c_filt2/1 -> Mux2/3
  Gain5/1 -> Simulink-PS Converter13/1
  n_load_machine/1 -> Gain7/1
  Gain9/1 -> Bus Creator/14  "omega_el"
  Impact Load without TMS/1 -> Simulink-PS Converter6/1
  Gain4/1 -> Voltages/3, Mux4/3  "u_c"
  voltage u_c_filt3/1 -> Mux2/2
  voltage u_b_filt1/1 -> 12bit ADC1/1(u)
  voltage u_c_filt1/1 -> 12bit ADC2/1(u)
  12bit ADC1/1(y) -> Gain3/1
  PWM | GPIO2/1 -> Simulink-PS Converter4/1
  Inner Torque/1 -> "Inner Torque "/1
  Demux4/3 -> Simulink-PS Converter10/1
  Bus Creator/1 -> ActualValues/1
  12bit ADC2/1(y) -> Gain4/1
  angle/1 -> Data Type Conversion1/1, Gain/1  "theta_m"
  PWM | GPIO/1 -> Simulink-PS Converter/1
  Data Type Conversion49/1 -> Simulink-PS Converter12/1
  Data Type Conversion5/1 -> Bus Creator/13, Gain9/1  "omega_m"
  PWM | GPIO3/1 -> Simulink-PS Converter1/1
  Demux4/1 -> Simulink-PS Converter8/1
  Saturation/1 -> Simulink-PS Converter7/1
  Demux4/2 -> Simulink-PS Converter9/1
  sensor noise2/1 -> Sum2/2
  voltage u_s/1 -> Data Type Conversion2/1  "V_DC"
  Ramp/1 -> Saturation/1
  Mux2/1 -> Rate Transition55/1
  voltage u_c_filt4/1 -> Mux2/1
  In Bus Element4/1 -> Rate Transition9/1
  Data Type Conversion48/1 -> PWM/1(In1), Switch5/3
  FOC_enabled/1 -> Switch5/2
  In Bus Element/1 -> Mux1/1
  In Bus Element3/1 -> Mux1/3
  In Bus Element2/1 -> Mux1/2
  PWM_FOC_in/1 -> Switch5/1
  Rate Transition45/1 -> Data Type Conversion48/1
  Data Type Conversion1/1 -> Sum4/1
  Rate Transition7/1 -> Switch2/2
  "0 = sinusoidal voltage source 1 = inverter    "/1 -> Switch2/3
  Rate Transition1/1 -> Switch3/2
  " "/1 -> Switch3/3, Switch2/1
  "   "/1 -> Switch3/1
  Switch3/1 -> Logical Operator1/1
  Switch2/1 -> Logical Operator1/2
  Data Type Conversion3/1 -> Simulink-PS Converter11/1
  Logical Operator1/1 -> Data Type Conversion3/1, Logical Operator/1
  In Bus Element10/1 -> Rate Transition1/1, Rate Transition7/1
  i_zero/1 -> Bus Creator4/3  "zero"
  Demux6/3 -> Bus Creator1/3  "c"
  v_q/1 -> Bus Creator3/2  "q"
  Demux6/2 -> Bus Creator1/2  "b"
  i_q/1 -> Bus Creator4/2  "q"
  Bus Creator3/1 -> Bus Creator/4  "v_dq"
  Demux6/1 -> Bus Creator1/1  "a"
  i_d/1 -> Bus Creator4/1  "d"
  v_d/1 -> Bus Creator3/1  "d"
  v_zero/1 -> Bus Creator3/3  "zero"
  Bus Creator4/1 -> Bus Creator/3  "i_dq"
  Bus Creator2/1 -> Bus Creator/2  "I_abc"
  Bus Creator1/1 -> Bus Creator/1  "V_abc"
  Demux8/1 -> Bus Creator2/1  "a"
  Demux8/2 -> Bus Creator2/2  "b"
  Demux8/3 -> Bus Creator2/3  "c"
  Gain6/1 -> Bus Creator/16  "theta_el"
  Constant/1 -> PWM | GPIO5/1, PWM | GPIO2/1, PWM | GPIO4/1, PWM | GPIO1/1, PWM | GPIO3/1, PWM | GPIO/1
  Mux4/1 -> Demux6/1  "V_UVW"
  In Bus Element6/1 -> Switch4/2
  Switch4/1 -> Sum4/2
  v_zero1/1 -> Switch4/3  "zero"
  In Bus Element5/1 -> Switch4/1
  Constant16/1 -> Demux2/1
  Constant17/1 -> Demux3/1
  Demux2/3 -> Bus Creator11/3, Bus Creator10/3  "c1"
  Demux2/1 -> Bus Creator11/1, Bus Creator10/1  "a1"
  Demux2/2 -> Bus Creator11/2, Bus Creator10/2  "b1"
  Demux3/2 -> Bus Creator11/5, Bus Creator10/5  "b2"
  Demux3/1 -> Bus Creator11/4, Bus Creator10/4  "a2"
  Demux3/3 -> Bus Creator11/6, Bus Creator10/6  "c2"
  Constant7/1 -> Bus Creator5/6, Bus Creator6/6  "z2"
  Constant3/1 -> Bus Creator5/3, Bus Creator6/3  "x"
  Constant4/1 -> Bus Creator5/4, Bus Creator6/4  "y"
  Constant1/1 -> Bus Creator5/1, Bus Creator6/1  "d"
  Constant2/1 -> Bus Creator5/2, Bus Creator6/2  "q"
  Constant5/1 -> Bus Creator5/5, Bus Creator6/5  "z1"
  Demux5/3 -> Bus Creator8/3  "zero"
  Demux10/2 -> Bus Creator12/2  "q"
  Demux7/3 -> Bus Creator7/3  "zero"
  Demux10/1 -> Bus Creator12/1  "d"
  Constant12/1 -> Demux10/1
  Demux5/1 -> Bus Creator8/1  "d"
  Demux9/3 -> Bus Creator9/3  "zero"
  Constant10/1 -> Demux7/1
  Demux9/2 -> Bus Creator9/2  "q"
  Demux10/3 -> Bus Creator12/3  "zero"
  Demux7/2 -> Bus Creator7/2  "q"
  Constant11/1 -> Demux9/1
  Demux7/1 -> Bus Creator7/1  "d"
  Constant9/1 -> Demux5/1
  Demux5/2 -> Bus Creator8/2  "q"
  Demux9/1 -> Bus Creator9/1  "d"
  Bus Creator10/1 -> Bus Creator/5  "v_abc_6ph"
  Bus Creator11/1 -> Bus Creator/6  "i_abc_6ph"
  Bus Creator8/1 -> Bus Creator/7  "v_xy_rotating"
  Bus Creator7/1 -> Bus Creator/8  "i_xy_rotating"
  Bus Creator9/1 -> Bus Creator/9  "v_zero_rotating"
  Bus Creator12/1 -> Bus Creator/10  "i_zero_rotating"
  Bus Creator6/1 -> Bus Creator/11  "i_dq_6ph"
  Bus Creator5/1 -> Bus Creator/12  "v_dq_6ph"
  Constant13/1 -> Bus Creator/18  "average_winding_temp"
  connections:
  Switch_0/RConn2 -- Switch1/LConn2 -- Switch_1/RConn1
  u_b_filt1/LConn1 -- 95,3kOhm4/LConn1 -- Permanent Magnet Synchronous Motor/LConn2 -- i_b/RConn2
  Switch f. TMS/RConn1 -- Measurement Shaft/LConn1
  Switch_4/RConn1 -- Switch_2/RConn1 -- v_DC/LConn1 -- V_DC/LConn1 -- Switch_0/RConn1
  Simulink-PS Converter8/RConn1 -- Controlled Voltage Source/RConn1
  47nF/RConn1 -- Controlled Voltage Source/RConn2 -- Controlled Voltage Source1/RConn2 -- Controlled Voltage Source2/RConn2 -- Electrical Reference/LConn1 -- Switch_5/RConn2 -- Switch_3/RConn2 -- Switch_1/RConn2 -- v_DC/RConn2 -- V_DC/RConn1 -- Solver Configuration/RConn1 -- u_b_filt/RConn2 -- 0.1µF1/RConn1 -- 4,99kOhm1/RConn1 -- u_b_filt1/RConn2 -- u_c_filt1/RConn2 -- u_a_filt1/RConn2 -- 4,99kOhm2/RConn1 -- 0.1µF2/RConn1 -- u_c_filt/RConn2 -- 8,2kOhm/RConn1 -- u_a_filt/RConn2
  Simulink-PS Converter6/RConn1 -- Ideal Torque Source/RConn1
  Load Friction/RConn1 -- Ideal Angular Velocity Source1/RConn2 -- Load Torque/RConn2 -- Motor Encoder/RConn1 -- Permanent Magnet Synchronous Motor/RConn2 -- Mechanical Rotational Reference/LConn1 -- Motor Friction/RConn1 -- Rotational Hard Stop/RConn1 -- Ideal Torque Source/RConn2 -- Ideal Angular Velocity Source/RConn2
  current b/LConn1 -- i_b/RConn1
  Coupling Encoder/LConn1 -- Ideal Torque Source/LConn1 -- Ideal Angular Velocity Source/LConn1 -- coupling m. shaft/LConn1 -- Motor Friction/LConn1 -- Rotational Hard Stop/LConn1 -- "Motor Inertia "/LConn1 -- Ideal Torque Sensor1/RConn1
  Switch_2/RConn2 -- Switch1/LConn3 -- Switch_3/RConn1
  u_c_filt/LConn1 -- 0.1µF2/LConn1 -- 4,99kOhm2/LConn1 -- 95,3kOhm5/RConn1
  voltage u_a_filt1/LConn1 -- u_a_filt/RConn1
  Simulink-PS Converter5/RConn1 -- Switch_5/LConn1
  Simulink-PS Converter/RConn1 -- Switch_0/LConn1
  voltage u_c_filt4/LConn1 -- u_a_filt1/RConn1
  Switch/LConn4 -- Controlled Voltage Source2/LConn1
  Switch_4/RConn2 -- Switch1/LConn4 -- Switch_5/RConn1
  Switch/RConn3 -- Switch1/RConn3 -- i_c/LConn1
  current c/LConn1 -- i_c/RConn1
  Simulink-PS Converter2/RConn1 -- Switch_2/LConn1
  Load Friction/LConn1 -- Ideal Torque Sensor/RConn1 -- Load Inertia/LConn1 -- Load Torque/LConn1 -- Ideal Angular Velocity Source1/LConn1
  current a/LConn1 -- i_a/RConn1
  speed/LConn1 -- Motor Encoder/RConn2
  voltage u_c_filt2/LConn1 -- u_c_filt1/RConn1
  Simulink-PS Converter1/RConn1 -- Switch_1/LConn1
  u_c_filt1/LConn1 -- 95,3kOhm5/LConn1 -- i_c/RConn2 -- Permanent Magnet Synchronous Motor/LConn3
  u_a_filt1/LConn1 -- 95,3kOhm/LConn1 -- i_a/RConn2 -- Permanent Magnet Synchronous Motor/LConn1
  Simulink-PS Converter10/RConn1 -- Controlled Voltage Source2/RConn1
  Coupling Encoder/RConn1 -- Encoder Inertia/LConn1 -- Motor Encoder/LConn1
  Switch/LConn2 -- Controlled Voltage Source/LConn1
  Switch/RConn1 -- Switch1/RConn1 -- i_a/LConn1
  Simulink-PS Converter9/RConn1 -- Controlled Voltage Source1/RConn1
  coupling m. shaft/RConn1 -- Switch f. TMS/LConn1
  Simulink-PS Converter11/RConn1 -- Switch1/LConn1
  Measurement Shaft/RConn1 -- Ideal Torque Sensor/LConn1
  Simulink-PS Converter12/RConn1 -- Switch/LConn1
  voltage u_s/LConn1 -- v_DC/RConn1
  Simulink-PS Converter13/RConn1 -- Load Torque/RConn1
  Open Circuit/LConn1 -- Permanent Magnet Synchronous Motor/LConn4
  Ideal Torque Sensor1/RConn2 -- Inner Torque/LConn1
  Simulink-PS Converter14/RConn1 -- Ideal Angular Velocity Source1/RConn1
  Ideal Torque Sensor1/LConn1 -- Permanent Magnet Synchronous Motor/RConn1
  voltage u_c_filt3/LConn1 -- u_b_filt1/RConn1
  Simulink-PS Converter4/RConn1 -- Switch_4/LConn1
  Switch/RConn2 -- Switch1/RConn2 -- i_b/LConn1
  voltage u_b_filt1/LConn1 -- u_b_filt/RConn1
  Simulink-PS Converter7/RConn1 -- Ideal Angular Velocity Source/RConn1
  u_a_filt/LConn1 -- 47nF/LConn1 -- 8,2kOhm/LConn1 -- 95,3kOhm/RConn1
  0.1µF1/LConn1 -- u_b_filt/LConn1 -- 4,99kOhm1/LConn1 -- 95,3kOhm4/RConn1
  voltage u_c_filt1/LConn1 -- u_c_filt/RConn1
  Torque M.shaft/LConn1 -- Ideal Torque Sensor/RConn2
  angle/LConn1 -- Motor Encoder/RConn3
  Switch/LConn3 -- Controlled Voltage Source1/LConn1
  Simulink-PS Converter3/RConn1 -- Switch_3/LConn1

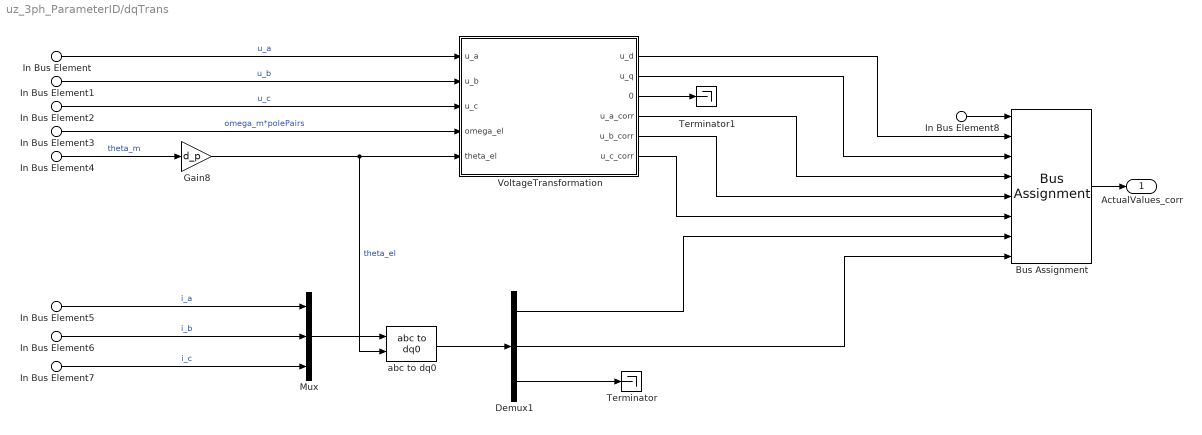
== system uz_3ph_ParameterID/dqTrans ==
  In Bus Element8 : Inport  PortName=ActualValues
  In Bus Element3 : Inport  PortName=ActualValues  Element=omega_el
  In Bus Element4 : Inport  PortName=ActualValues  Element=theta_m
  In Bus Element : Inport  PortName=ActualValues  Element=V_abc.a
  In Bus Element1 : Inport  PortName=ActualValues  Element=V_abc.b
  In Bus Element2 : Inport  PortName=ActualValues  Element=V_abc.c
  In Bus Element5 : Inport  PortName=ActualValues  Element=I_abc.a
  In Bus Element6 : Inport  PortName=ActualValues  Element=I_abc.b
  In Bus Element7 : Inport  PortName=ActualValues  Element=I_abc.c
  Bus Assignment : BusAssignment  AssignedSignals=v_dq.d,v_dq.q,V_abc.a,V_abc.b,V_abc.c,i_dq.d,i_dq.q
  Demux1 : Demux  Outputs=3
  Gain8 : Gain  Gain=d_p  OutDataTypeStr=single
  Mux : Mux  Inputs=3
  Terminator : Terminator
  Terminator1 : Terminator
  VoltageTransformation : Subsystem
  abc to dq0 : spsabctodq0Lib/abc to dq0  Alignment=Aligned with phase A axis
  ActualValues_corr : Outport  OutDataTypeStr=Bus: uz_ParaID_ActualValues_t
  wires:
  VoltageTransformation/3(0) -> Terminator1/1
  In Bus Element3/1 -> VoltageTransformation/4(omega_el)  "omega_m*polePairs"
  In Bus Element2/1 -> VoltageTransformation/3(u_c)  "u_c"
  In Bus Element1/1 -> VoltageTransformation/2(u_b)  "u_b"
  In Bus Element/1 -> VoltageTransformation/1(u_a)  "u_a"
  Demux1/3 -> Terminator/1
  Mux/1 -> abc to dq0/1
  In Bus Element7/1 -> Mux/3  "i_c"
  In Bus Element6/1 -> Mux/2  "i_b"
  In Bus Element5/1 -> Mux/1  "i_a"
  Demux1/2 -> Bus Assignment/8
  Demux1/1 -> Bus Assignment/7
  abc to dq0/1 -> Demux1/1
  VoltageTransformation/2(u_q) -> Bus Assignment/3
  VoltageTransformation/1(u_d) -> Bus Assignment/2
  VoltageTransformation/4(u_a_corr) -> Bus Assignment/4
  VoltageTransformation/5(u_b_corr) -> Bus Assignment/5
  VoltageTransformation/6(u_c_corr) -> Bus Assignment/6
  In Bus Element8/1 -> Bus Assignment/1
  Bus Assignment/1 -> ActualValues_corr/1
  Gain8/1 -> abc to dq0/2, VoltageTransformation/5(theta_el)  "theta_el"
  In Bus Element4/1 -> Gain8/1  "theta_m"
